simulink model "Droop_GC"  (Simulink 9.1)
settings: Solver=ode4  StartTime=0.0  StopTime=2.6  FixedStep=1e-6  RelTol=1e-3  EnableMultiTasking=on
InitFcn:
  | %% Circuit parameters
  | % LC filter
  | Lf_1 = 1.35e-3;
  | Rf_1 = 0.1;
  | Cf_1 = 50e-6;
  | 
  | Lf_2 = 1.35e-3;
  | Rf_2 = 0.1;
  | Cf_2 = 50e-6;
  | 
  | Lf_3 = 1.35e-3;
  | Rf_3 = 0.1;
  | Cf_3 = 50e-6;
  | 
  | % transmission line(grid coupling impedance)
  | L_1 = 0.35e-3;
  | R_1 = 0.03;
  | 
  | L_2 = 0.35e-3;
  | R_2 = 0.03;
  | 
  | L_3 = 0.35e-3;
  | R_3 = 0.03;
  | 
  | % Network
  | % active power loop
  | fn = 50;
  | wn = 2*pi*fn;
  | 
  | R_line_1 = 0.23;
  | L_line_1 = 0.1 / wn;
  | 
  | R_line_2 = 0.35;
  | L_line_2 = 0.58 / wn;
  | 
  | 
  | %% Control parameters
  | % power measurement LPF
  | wc = 31.41;
  | 
  | % Power droop
  | mp_1 = mp;
  | mp_2 = mp;
  | mp_3 = mp;
  | 
  | nq_1 = nq;
  | nq_2 = nq;
  | nq_3 = nq;
  | 
  | J1 = 0.1;
  | J2 = 0.1;
  | J3 = 0.1;
  | 
  | Pref_1 = Pref;
  | Pref_2 = Pref;
  | Pref_3 = Pref;
  | 
  | % outer voltage loop
  | Kpv_1 = 0.05;
  | Kiv_1 = 390;
  | ... (+76 lines)
values from neighbouring files (symbols this model uses):
  mp = 9.4e-5    (= 9.4e-05)    [model_coefficient.m]
  nq = 1.3e-3    (= 0.0013)    [model_coefficient.m]
  Pref = 10000    [model_coefficient.m]
  R1 = 25    [model_coefficient.m]
  R3 = 20    [model_coefficient.m]
libraries: powerlib x53, powerlib_meascontrol x25
(part 2 of 2)

== system Droop_GC/sm_computation/VSI 1/1_VSG control block/SRF PLL1 ==
  Vg_abc : Inport
  Demux2 : Demux  Outputs=3
  LPF2 : TransferFcn  Numerator=[wf_pll]  Denominator=[1 wf_pll]
  SRF_PLL : Subsystem
  Tclark : Subsystem
  Tpark : Subsystem
  Vg_theta : Outport
  wires:
  Demux2/1 -> Tclark/1(Ua)
  Demux2/2 -> Tclark/2(Ub)
  Demux2/3 -> Tclark/3(Uc)
  Tclark/1(Valpha) -> Tpark/1(Ualpha)
  Tpark/2(Uq) -> LPF2/1
  LPF2/1 -> SRF_PLL/1(vq)  "SRF_vq"
  Vg_abc/1 -> Demux2/1
  Tclark/2(Vbeta) -> Tpark/2(Ubeta)
  SRF_PLL/1(wt) -> Tpark/3(theta), Vg_theta/1  "SRF_wt_mod"

== system Droop_GC/sm_computation/VSI 1/1_VSG control block/Subsystem ==
  theta_g : Inport
  Enable_sync : Inport  Port=2
  theta_vsg : Inport  Port=3
  Add : Sum  Inputs=-+
  Constant : Constant  Value=0
  Gain : Gain  Gain=Kp_syn
  Gain1 : Gain  Gain=Ki_syn
  Integrator2 : Integrator
  Sum2 : Sum  Inputs=|++
  Switch : Switch  Criteria=u2 > Threshold
  delta_w : Outport
  wires:
  Gain1/1 -> Integrator2/1
  Integrator2/1 -> Sum2/2
  Sum2/1 -> Switch/1
  Add/1 -> Gain1/1, Gain/1
  Gain/1 -> Sum2/1
  theta_g/1 -> Add/2
  theta_vsg/1 -> Add/1
  Switch/1 -> delta_w/1
  Enable_sync/1 -> Switch/2
  Constant/1 -> Switch/3

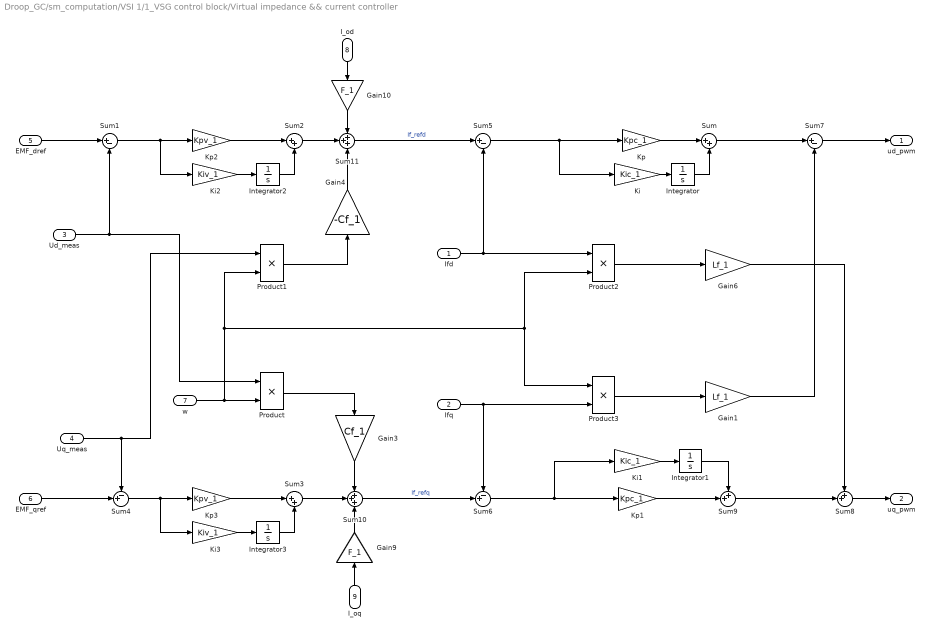
== system Droop_GC/sm_computation/VSI 1/1_VSG control block/Virtual impedance && current controller ==
  Ifd : Inport
  Ifq : Inport  Port=2
  Ud_meas : Inport  Port=3
  Uq_meas : Inport  Port=4
  EMF_dref : Inport  Port=5
  EMF_qref : Inport  Port=6
  w : Inport  Port=7
  I_od : Inport  Port=8
  I_oq : Inport  Port=9
  Gain1 : Gain  Gain=Lf_1
  Gain10 : Gain  Gain=F_1
  Gain3 : Gain  Gain=Cf_1
  Gain4 : Gain  Gain=-Cf_1
  Gain6 : Gain  Gain=Lf_1
  Gain9 : Gain  Gain=F_1
  Integrator{,1..3} (4 alike) : Integrator
  Ki : Gain  Gain=Kic_1
  Ki1 : Gain  Gain=Kic_1
  Ki2 : Gain  Gain=Kiv_1
  Ki3 : Gain  Gain=Kiv_1
  Kp : Gain  Gain=Kpc_1
  Kp1 : Gain  Gain=Kpc_1
  Kp2 : Gain  Gain=Kpv_1
  Kp3 : Gain  Gain=Kpv_1
  Product{,1..3} (4 alike) : Product
  Sum : Sum  Inputs=|++
  Sum1 : Sum  Inputs=|+-
  Sum10 : Sum  Inputs=+++
  Sum11 : Sum  Inputs=+++
  Sum2 : Sum  Inputs=|++
  Sum3 : Sum  Inputs=|++
  Sum4 : Sum  Inputs=-+|
  Sum5 : Sum  Inputs=|+-
  Sum6 : Sum  Inputs=-+|
  Sum7 : Sum  Inputs=|+-
  Sum8 : Sum  Inputs=++|
  Sum9 : Sum  Inputs=++|
  ud_pwm : Outport
  uq_pwm : Outport  Port=2
  wires:
  Sum7/1 -> ud_pwm/1
  Ifd/1 -> Sum5/2, Product2/1
  Ifq/1 -> Product3/2, Sum6/1
  Ki/1 -> Integrator/1
  Kp/1 -> Sum/1
  Integrator/1 -> Sum/2
  Sum11/1 -> Sum5/1  "If_refd"
  Sum10/1 -> Sum6/2  "If_refq"
  Sum8/1 -> uq_pwm/1
  Ki1/1 -> Integrator1/1
  Sum9/1 -> Sum8/2
  Sum5/1 -> Ki/1, Kp/1
  Kp1/1 -> Sum9/2
  Integrator1/1 -> Sum9/1
  Sum6/1 -> Ki1/1, Kp1/1
  EMF_dref/1 -> Sum1/1
  Ud_meas/1 -> Sum1/2, Product/1
  EMF_qref/1 -> Sum4/2
  Uq_meas/1 -> Product1/1, Sum4/1
  Sum1/1 -> Ki2/1, Kp2/1
  Integrator2/1 -> Sum2/2
  Kp2/1 -> Sum2/1
  Ki2/1 -> Integrator2/1
  Ki3/1 -> Integrator3/1
  Kp3/1 -> Sum3/1
  Sum4/1 -> Ki3/1, Kp3/1
  Integrator3/1 -> Sum3/2
  w/1 -> Product3/1, Product2/2, Product1/2, Product/2
  Product/1 -> Gain3/1
  Sum3/1 -> Sum10/2
  Gain3/1 -> Sum10/1
  Product1/1 -> Gain4/1
  Sum2/1 -> Sum11/2
  Gain4/1 -> Sum11/3
  I_oq/1 -> Gain9/1
  Gain9/1 -> Sum10/3
  I_od/1 -> Gain10/1
  Gain10/1 -> Sum11/1
  Sum/1 -> Sum7/1
  Product2/1 -> Gain6/1
  Gain6/1 -> Sum8/1
  Product3/1 -> Gain1/1
  Gain1/1 -> Sum7/2

== system Droop_GC/sm_computation/VSI 1/1_VSG control block/active power controller ==
  Pe : Inport
  delta_w : Inport  Port=2
  Constant : Constant  Value=wn
  Gain2 : Gain  Gain=mp_1
  Integrator3 : Integrator
  Pref_INV1 : Constant  Value=Pref_1
  Sum2 : Sum  Inputs=|++
  Sum3 : Sum  Inputs=+-
  Sum6 : Sum  Inputs=++|
  theta : Outport
  w : Outport  Port=2
  wires:
  Pe/1 -> Sum3/2
  Pref_INV1/1 -> Sum3/1
  Sum3/1 -> Gain2/1
  Constant/1 -> Sum6/2
  Gain2/1 -> Sum6/1
  delta_w/1 -> Sum2/2
  Sum6/1 -> Sum2/1  "w"
  Sum2/1 -> w/1, Integrator3/1
  Integrator3/1 -> theta/1

== system Droop_GC/sm_computation/VSI 1/1_VSG control block/reactive power controller ==
  Qe : Inport
  Dq_1 : Gain  Gain=nq_1
  Sum1 : Sum  Inputs=|+-
  Vn1 : Constant  Value=sqrt(2)*V_phase_rms
  Em : Outport
  wires:
  Sum1/1 -> Em/1  "delta_P"
  Qe/1 -> Dq_1/1
  Dq_1/1 -> Sum1/2
  Vn1/1 -> Sum1/1

== system Droop_GC/sm_computation/VSI 2/1_VSG control block/Power Calculation ==
  note: Iabc
  note: Vabc
  Vin : Inport
  Iin : Inport  Port=2
  Add : Sum
  Add1 : Sum  Inputs=-+
  Demux1 : Demux  Outputs=3
  Demux2 : Demux  Outputs=3
  Gain1 : Gain  Gain=3/2
  Gain2 : Gain  Gain=3/2
  Product{,1..3} (4 alike) : Product
  Terminator : Terminator
  Terminator1 : Terminator
  abc to Alpha-Beta-Zero : powerlib_meascontrol/Transformations/abc to Alpha-Beta-Zero
      settings: SourceProductName=Simscape Power Systems
  abc to Alpha-Beta-Zero1 : powerlib_meascontrol/Transformations/abc to Alpha-Beta-Zero
      settings: SourceProductName=Simscape Power Systems
  P : Outport
  Q : Outport  Port=2
  wires:
  Add1/1 -> Gain1/1
  Add/1 -> Gain2/1
  Demux2/2 -> Product1/2, Product2/2
  Product3/1 -> Add1/2
  Product2/1 -> Add1/1
  Product1/1 -> Add/2
  Product/1 -> Add/1
  abc to Alpha-Beta-Zero/1 -> Demux1/1
  Demux1/1 -> Product2/1, Product/1
  abc to Alpha-Beta-Zero1/1 -> Demux2/1
  Demux2/3 -> Terminator1/1
  Demux1/3 -> Terminator/1
  Demux2/1 -> Product3/2, Product/2
  Demux1/2 -> Product3/1, Product1/1
  Vin/1 -> abc to Alpha-Beta-Zero/1
  Iin/1 -> abc to Alpha-Beta-Zero1/1
  Gain2/1 -> P/1
  Gain1/1 -> Q/1

== system Droop_GC/sm_computation/VSI 2/1_VSG control block/SRF PLL ==
  Vg_abc : Inport
  Demux2 : Demux  Outputs=3
  LPF2 : TransferFcn  Numerator=[wf_pll]  Denominator=[1 wf_pll]
  LPF3 : TransferFcn  Numerator=[wf_pll]  Denominator=[1 wf_pll]
  SRF_PLL : Subsystem
  Tclark : Subsystem
  Tpark : Subsystem
  Vg_theta : Outport
  wires:
  Demux2/1 -> Tclark/1(Ua)
  Demux2/2 -> Tclark/2(Ub)
  Demux2/3 -> Tclark/3(Uc)
  Tpark/1(Ud) -> LPF3/1
  Tclark/1(Valpha) -> Tpark/1(Ualpha)
  Tpark/2(Uq) -> LPF2/1
  LPF2/1 -> SRF_PLL/1(vq)  "SRF_vq"
  Vg_abc/1 -> Demux2/1
  Tclark/2(Vbeta) -> Tpark/2(Ubeta)
  SRF_PLL/1(wt) -> Tpark/3(theta), Vg_theta/1  "SRF_wt_mod"

== system Droop_GC/sm_computation/VSI 2/1_VSG control block/SRF PLL1 ==
  Vg_abc : Inport
  Demux2 : Demux  Outputs=3
  LPF2 : TransferFcn  Numerator=[wf_pll]  Denominator=[1 wf_pll]
  SRF_PLL : Subsystem
  Tclark : Subsystem
  Tpark : Subsystem
  Vg_theta : Outport
  wires:
  Demux2/1 -> Tclark/1(Ua)
  Demux2/2 -> Tclark/2(Ub)
  Demux2/3 -> Tclark/3(Uc)
  Tclark/1(Valpha) -> Tpark/1(Ualpha)
  Tpark/2(Uq) -> LPF2/1
  LPF2/1 -> SRF_PLL/1(vq)  "SRF_vq"
  Vg_abc/1 -> Demux2/1
  Tclark/2(Vbeta) -> Tpark/2(Ubeta)
  SRF_PLL/1(wt) -> Tpark/3(theta), Vg_theta/1  "SRF_wt_mod"

== system Droop_GC/sm_computation/VSI 2/1_VSG control block/Subsystem ==
  theta_g : Inport
  Enable_sync : Inport  Port=2
  theta_vsg : Inport  Port=3
  Add : Sum  Inputs=-+
  Constant : Constant  Value=0
  Gain : Gain  Gain=Kp_syn
  Gain1 : Gain  Gain=Ki_syn
  Integrator2 : Integrator
  Sum2 : Sum  Inputs=|++
  Switch : Switch  Criteria=u2 > Threshold
  delta_w : Outport
  wires:
  Gain1/1 -> Integrator2/1
  Integrator2/1 -> Sum2/2
  Sum2/1 -> Switch/1
  Add/1 -> Gain1/1, Gain/1
  Gain/1 -> Sum2/1
  theta_g/1 -> Add/2
  theta_vsg/1 -> Add/1
  Switch/1 -> delta_w/1
  Enable_sync/1 -> Switch/2
  Constant/1 -> Switch/3

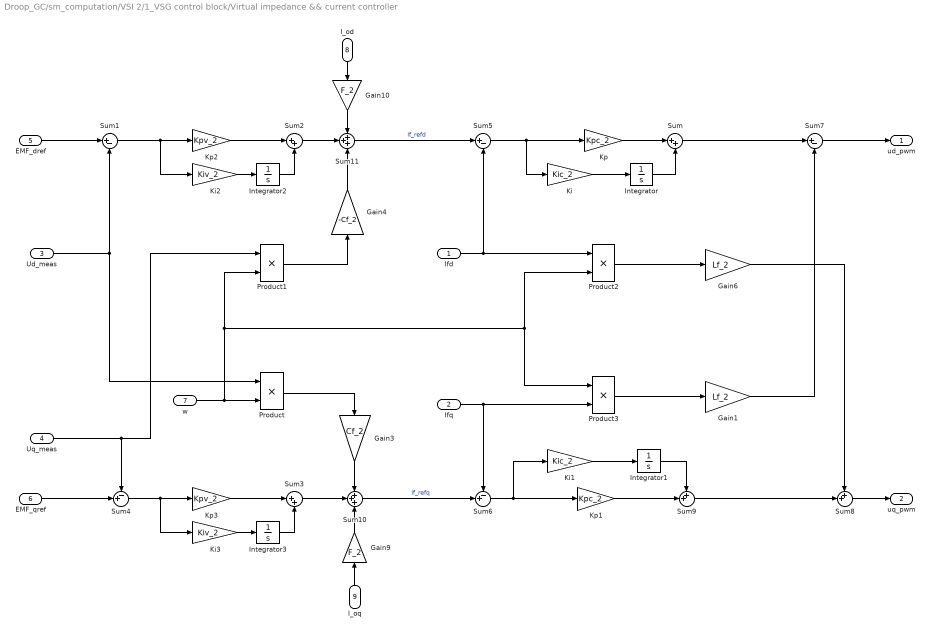
== system Droop_GC/sm_computation/VSI 2/1_VSG control block/Virtual impedance && current controller ==
  Ifd : Inport
  Ifq : Inport  Port=2
  Ud_meas : Inport  Port=3
  Uq_meas : Inport  Port=4
  EMF_dref : Inport  Port=5
  EMF_qref : Inport  Port=6
  w : Inport  Port=7
  I_od : Inport  Port=8
  I_oq : Inport  Port=9
  Gain1 : Gain  Gain=Lf_2
  Gain10 : Gain  Gain=F_2
  Gain3 : Gain  Gain=Cf_2
  Gain4 : Gain  Gain=-Cf_2
  Gain6 : Gain  Gain=Lf_2
  Gain9 : Gain  Gain=F_2
  Integrator{,1..3} (4 alike) : Integrator
  Ki : Gain  Gain=Kic_2
  Ki1 : Gain  Gain=Kic_2
  Ki2 : Gain  Gain=Kiv_2
  Ki3 : Gain  Gain=Kiv_2
  Kp : Gain  Gain=Kpc_2
  Kp1 : Gain  Gain=Kpc_2
  Kp2 : Gain  Gain=Kpv_2
  Kp3 : Gain  Gain=Kpv_2
  Product{,1..3} (4 alike) : Product
  Sum : Sum  Inputs=|++
  Sum1 : Sum  Inputs=|+-
  Sum10 : Sum  Inputs=+++
  Sum11 : Sum  Inputs=+++
  Sum2 : Sum  Inputs=|++
  Sum3 : Sum  Inputs=|++
  Sum4 : Sum  Inputs=-+|
  Sum5 : Sum  Inputs=|+-
  Sum6 : Sum  Inputs=-+|
  Sum7 : Sum  Inputs=|+-
  Sum8 : Sum  Inputs=++|
  Sum9 : Sum  Inputs=++|
  ud_pwm : Outport
  uq_pwm : Outport  Port=2
  wires:
  Gain1/1 -> Sum7/2
  Product3/1 -> Gain1/1
  Gain6/1 -> Sum8/1
  Product2/1 -> Gain6/1
  Sum/1 -> Sum7/1
  Gain10/1 -> Sum11/1
  I_od/1 -> Gain10/1
  Gain9/1 -> Sum10/3
  I_oq/1 -> Gain9/1
  Gain4/1 -> Sum11/3
  Sum2/1 -> Sum11/2
  Product1/1 -> Gain4/1
  Gain3/1 -> Sum10/1
  Sum3/1 -> Sum10/2
  Product/1 -> Gain3/1
  w/1 -> Product/2, Product1/2, Product2/2, Product3/1
  Integrator3/1 -> Sum3/2
  Sum4/1 -> Kp3/1, Ki3/1
  Kp3/1 -> Sum3/1
  Ki3/1 -> Integrator3/1
  Ki2/1 -> Integrator2/1
  Kp2/1 -> Sum2/1
  Integrator2/1 -> Sum2/2
  Sum1/1 -> Kp2/1, Ki2/1
  Uq_meas/1 -> Product1/1, Sum4/1
  EMF_qref/1 -> Sum4/2
  Ud_meas/1 -> Product/1, Sum1/2
  EMF_dref/1 -> Sum1/1
  Sum6/1 -> Kp1/1, Ki1/1
  Integrator1/1 -> Sum9/1
  Kp1/1 -> Sum9/2
  Sum5/1 -> Kp/1, Ki/1
  Sum9/1 -> Sum8/2
  Ki1/1 -> Integrator1/1
  Sum8/1 -> uq_pwm/1
  Sum10/1 -> Sum6/2  "If_refq"
  Sum11/1 -> Sum5/1  "If_refd"
  Integrator/1 -> Sum/2
  Kp/1 -> Sum/1
  Ki/1 -> Integrator/1
  Ifq/1 -> Sum6/1, Product3/2
  Ifd/1 -> Product2/1, Sum5/2
  Sum7/1 -> ud_pwm/1

== system Droop_GC/sm_computation/VSI 2/1_VSG control block/active power controller ==
  Pe : Inport
  delta_w : Inport  Port=2
  Constant : Constant  Value=wn
  Gain1 : Gain  Gain=mp_2
  Integrator1 : Integrator
  Pref_INV2 : Constant  Value=Pref_2
  Sum1 : Sum  Inputs=++|
  Sum2 : Sum  Inputs=|++
  Sum3 : Sum  Inputs=|+-
  theta : Outport
  w : Outport  Port=2
  wires:
  Pref_INV2/1 -> Sum3/1
  Pe/1 -> Sum3/2
  Integrator1/1 -> theta/1
  delta_w/1 -> Sum2/2
  Sum2/1 -> w/1, Integrator1/1
  Sum3/1 -> Gain1/1
  Gain1/1 -> Sum1/1
  Constant/1 -> Sum1/2
  Sum1/1 -> Sum2/1

== system Droop_GC/sm_computation/VSI 2/1_VSG control block/reactive power controller ==
  Qe : Inport
  Dq_2 : Gain  Gain=nq_2
  Sum1 : Sum  Inputs=|+-
  Vn1 : Constant  Value=sqrt(2)*V_phase_rms
  Em : Outport
  wires:
  Vn1/1 -> Sum1/1
  Dq_2/1 -> Sum1/2
  Qe/1 -> Dq_2/1
  Sum1/1 -> Em/1  "delta_P"

== system Droop_GC/sm_computation/VSI 3/1_VSG control block/Power Calculation ==
  note: Iabc
  note: Vabc
  Vin : Inport
  Iin : Inport  Port=2
  Add : Sum
  Add1 : Sum  Inputs=-+
  Demux1 : Demux  Outputs=3
  Demux2 : Demux  Outputs=3
  Gain1 : Gain  Gain=3/2
  Gain2 : Gain  Gain=3/2
  Product{,1..3} (4 alike) : Product
  Terminator : Terminator
  Terminator1 : Terminator
  abc to Alpha-Beta-Zero : powerlib_meascontrol/Transformations/abc to Alpha-Beta-Zero
      settings: SourceProductName=Simscape Power Systems
  abc to Alpha-Beta-Zero1 : powerlib_meascontrol/Transformations/abc to Alpha-Beta-Zero
      settings: SourceProductName=Simscape Power Systems
  P : Outport
  Q : Outport  Port=2
  wires:
  Add1/1 -> Gain1/1
  Add/1 -> Gain2/1
  Demux2/2 -> Product1/2, Product2/2
  Product3/1 -> Add1/2
  Product2/1 -> Add1/1
  Product1/1 -> Add/2
  Product/1 -> Add/1
  abc to Alpha-Beta-Zero/1 -> Demux1/1
  Demux1/1 -> Product2/1, Product/1
  abc to Alpha-Beta-Zero1/1 -> Demux2/1
  Demux2/3 -> Terminator1/1
  Demux1/3 -> Terminator/1
  Demux2/1 -> Product3/2, Product/2
  Demux1/2 -> Product3/1, Product1/1
  Vin/1 -> abc to Alpha-Beta-Zero/1
  Iin/1 -> abc to Alpha-Beta-Zero1/1
  Gain2/1 -> P/1
  Gain1/1 -> Q/1

== system Droop_GC/sm_computation/VSI 3/1_VSG control block/SRF PLL ==
  Vg_abc : Inport
  Demux2 : Demux  Outputs=3
  LPF2 : TransferFcn  Numerator=[wf_pll]  Denominator=[1 wf_pll]
  LPF3 : TransferFcn  Numerator=[wf_pll]  Denominator=[1 wf_pll]
  SRF_PLL : Subsystem
  Tclark : Subsystem
  Tpark : Subsystem
  Vg_theta : Outport
  wires:
  Demux2/1 -> Tclark/1(Ua)
  Demux2/2 -> Tclark/2(Ub)
  Demux2/3 -> Tclark/3(Uc)
  Tpark/1(Ud) -> LPF3/1
  Tclark/1(Valpha) -> Tpark/1(Ualpha)
  Tpark/2(Uq) -> LPF2/1
  LPF2/1 -> SRF_PLL/1(vq)  "SRF_vq"
  Vg_abc/1 -> Demux2/1
  Tclark/2(Vbeta) -> Tpark/2(Ubeta)
  SRF_PLL/1(wt) -> Tpark/3(theta), Vg_theta/1  "SRF_wt_mod"

== system Droop_GC/sm_computation/VSI 3/1_VSG control block/SRF PLL1 ==
  Vg_abc : Inport
  Demux2 : Demux  Outputs=3
  LPF2 : TransferFcn  Numerator=[wf_pll]  Denominator=[1 wf_pll]
  SRF_PLL : Subsystem
  Tclark : Subsystem
  Tpark : Subsystem
  Vg_theta : Outport
  wires:
  Demux2/1 -> Tclark/1(Ua)
  Demux2/2 -> Tclark/2(Ub)
  Demux2/3 -> Tclark/3(Uc)
  Tclark/1(Valpha) -> Tpark/1(Ualpha)
  Tpark/2(Uq) -> LPF2/1
  LPF2/1 -> SRF_PLL/1(vq)  "SRF_vq"
  Vg_abc/1 -> Demux2/1
  Tclark/2(Vbeta) -> Tpark/2(Ubeta)
  SRF_PLL/1(wt) -> Tpark/3(theta), Vg_theta/1  "SRF_wt_mod"

== system Droop_GC/sm_computation/VSI 3/1_VSG control block/Subsystem ==
  theta_g : Inport
  Enable_sync : Inport  Port=2
  theta_vsg : Inport  Port=3
  Add : Sum  Inputs=-+
  Constant : Constant  Value=0
  Gain : Gain  Gain=Kp_syn
  Gain1 : Gain  Gain=Ki_syn
  Integrator2 : Integrator
  Sum2 : Sum  Inputs=|++
  Switch : Switch  Criteria=u2 > Threshold
  delta_w : Outport
  wires:
  Gain1/1 -> Integrator2/1
  Integrator2/1 -> Sum2/2
  Sum2/1 -> Switch/1
  Add/1 -> Gain1/1, Gain/1
  Gain/1 -> Sum2/1
  theta_g/1 -> Add/2
  theta_vsg/1 -> Add/1
  Switch/1 -> delta_w/1
  Enable_sync/1 -> Switch/2
  Constant/1 -> Switch/3

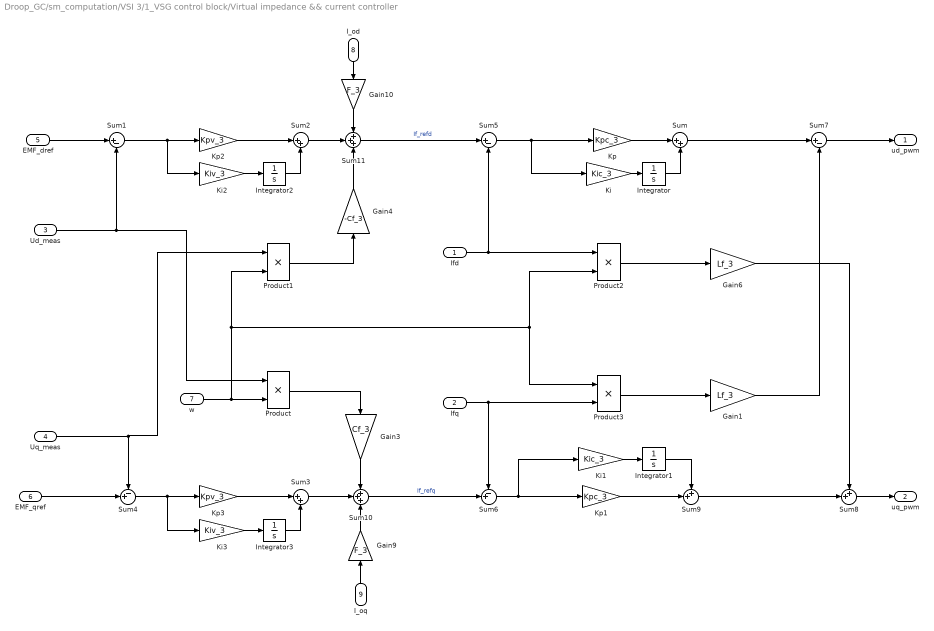
== system Droop_GC/sm_computation/VSI 3/1_VSG control block/Virtual impedance && current controller ==
  Ifd : Inport
  Ifq : Inport  Port=2
  Ud_meas : Inport  Port=3
  Uq_meas : Inport  Port=4
  EMF_dref : Inport  Port=5
  EMF_qref : Inport  Port=6
  w : Inport  Port=7
  I_od : Inport  Port=8
  I_oq : Inport  Port=9
  Gain1 : Gain  Gain=Lf_3
  Gain10 : Gain  Gain=F_3
  Gain3 : Gain  Gain=Cf_3
  Gain4 : Gain  Gain=-Cf_3
  Gain6 : Gain  Gain=Lf_3
  Gain9 : Gain  Gain=F_3
  Integrator{,1..3} (4 alike) : Integrator
  Ki : Gain  Gain=Kic_3
  Ki1 : Gain  Gain=Kic_3
  Ki2 : Gain  Gain=Kiv_3
  Ki3 : Gain  Gain=Kiv_3
  Kp : Gain  Gain=Kpc_3
  Kp1 : Gain  Gain=Kpc_3
  Kp2 : Gain  Gain=Kpv_3
  Kp3 : Gain  Gain=Kpv_3
  Product{,1..3} (4 alike) : Product
  Sum : Sum  Inputs=|++
  Sum1 : Sum  Inputs=|+-
  Sum10 : Sum  Inputs=+++
  Sum11 : Sum  Inputs=+++
  Sum2 : Sum  Inputs=|++
  Sum3 : Sum  Inputs=|++
  Sum4 : Sum  Inputs=-+|
  Sum5 : Sum  Inputs=|+-
  Sum6 : Sum  Inputs=-+|
  Sum7 : Sum  Inputs=|+-
  Sum8 : Sum  Inputs=++|
  Sum9 : Sum  Inputs=++|
  ud_pwm : Outport
  uq_pwm : Outport  Port=2
  wires:
  Sum7/1 -> ud_pwm/1
  Ifd/1 -> Sum5/2, Product2/1
  Ifq/1 -> Product3/2, Sum6/1
  Ki/1 -> Integrator/1
  Kp/1 -> Sum/1
  Integrator/1 -> Sum/2
  Sum11/1 -> Sum5/1  "If_refd"
  Sum10/1 -> Sum6/2  "If_refq"
  Sum8/1 -> uq_pwm/1
  Ki1/1 -> Integrator1/1
  Sum9/1 -> Sum8/2
  Sum5/1 -> Ki/1, Kp/1
  Kp1/1 -> Sum9/2
  Integrator1/1 -> Sum9/1
  Sum6/1 -> Ki1/1, Kp1/1
  EMF_dref/1 -> Sum1/1
  Ud_meas/1 -> Sum1/2, Product/1
  EMF_qref/1 -> Sum4/2
  Uq_meas/1 -> Product1/1, Sum4/1
  Sum1/1 -> Ki2/1, Kp2/1
  Integrator2/1 -> Sum2/2
  Kp2/1 -> Sum2/1
  Ki2/1 -> Integrator2/1
  Ki3/1 -> Integrator3/1
  Kp3/1 -> Sum3/1
  Sum4/1 -> Ki3/1, Kp3/1
  Integrator3/1 -> Sum3/2
  w/1 -> Product3/1, Product2/2, Product1/2, Product/2
  Product/1 -> Gain3/1
  Sum3/1 -> Sum10/2
  Gain3/1 -> Sum10/1
  Product1/1 -> Gain4/1
  Sum2/1 -> Sum11/2
  Gain4/1 -> Sum11/3
  I_oq/1 -> Gain9/1
  Gain9/1 -> Sum10/3
  I_od/1 -> Gain10/1
  Gain10/1 -> Sum11/1
  Sum/1 -> Sum7/1
  Product2/1 -> Gain6/1
  Gain6/1 -> Sum8/1
  Product3/1 -> Gain1/1
  Gain1/1 -> Sum7/2

== system Droop_GC/sm_computation/VSI 3/1_VSG control block/active power controller ==
  Pe : Inport
  delta_w : Inport  Port=2
  Constant : Constant  Value=wn
  Gain1 : Gain  Gain=mp_3
  Integrator1 : Integrator
  Pref_INV3 : Constant  Value=Pref_3
  Sum1 : Sum  Inputs=++|
  Sum2 : Sum  Inputs=|+-
  Sum3 : Sum  Inputs=|++
  theta : Outport
  w : Outport  Port=2
  wires:
  Pe/1 -> Sum2/2
  Pref_INV3/1 -> Sum2/1
  Integrator1/1 -> theta/1
  delta_w/1 -> Sum3/2
  Sum3/1 -> w/1, Integrator1/1
  Sum2/1 -> Gain1/1
  Constant/1 -> Sum1/2
  Gain1/1 -> Sum1/1
  Sum1/1 -> Sum3/1  "w"

== system Droop_GC/sm_computation/VSI 3/1_VSG control block/reactive power controller ==
  Qe : Inport
  Dq_3 : Gain  Gain=nq_3
  Sum1 : Sum  Inputs=|+-
  Vn1 : Constant  Value=sqrt(2)*V_phase_rms
  Em : Outport
  wires:
  Sum1/1 -> Em/1  "delta_P"
  Qe/1 -> Dq_3/1
  Dq_3/1 -> Sum1/2
  Vn1/1 -> Sum1/1

== system Droop_GC/sm_computation/VSI 1/1_VSG control block/SRF PLL/SRF_PLL ==
  vq : Inport
  Center_Fre : Constant  Value=wn
  Center_Fre1 : Constant  Value=220*sqrt(2)
  Divide : Product  Inputs=*/
  Integrator : Integrator
  Integrator1 : Integrator
  Ki : Gain  Gain=Ki_pll
  Kp : Gain  Gain=Kp_pll
  Sum : Sum  Inputs=|++
  Sum1 : Sum  Inputs=++|
  wt : Outport
  wires:
  Divide/1 -> Ki/1, Kp/1
  Kp/1 -> Sum/1
  Ki/1 -> Integrator/1
  Integrator/1 -> Sum/2
  Sum/1 -> Sum1/2
  Sum1/1 -> Integrator1/1
  Integrator1/1 -> wt/1
  vq/1 -> Divide/1
  Center_Fre/1 -> Sum1/1
  Center_Fre1/1 -> Divide/2

== system Droop_GC/sm_computation/VSI 1/1_VSG control block/SRF PLL/Tclark ==
  Ua : Inport
  Ub : Inport  Port=2
  Uc : Inport  Port=3
  Constant : Constant  Value=2/3
  Constant1 : Constant  Value=-1/3
  Constant2 : Constant  Value=-1/3
  Constant3 : Constant  Value=1/sqrt(3)
  Constant4 : Constant  Value=-1/sqrt(3)
  Product{,1..4} (5 alike) : Product
  Sum : Sum  Inputs=+++
  Sum1 : Sum
  Valpha : Outport
  Vbeta : Outport  Port=2
  wires:
  Product/1 -> Sum/1
  Constant1/1 -> Product1/1
  Product2/1 -> Sum/3
  Ua/1 -> Product/2
  Constant4/1 -> Product4/2
  Constant2/1 -> Product2/1
  Uc/1 -> Product4/1, Product2/2
  Constant/1 -> Product/1
  Sum/1 -> Valpha/1
  Product1/1 -> Sum/2
  Constant3/1 -> Product3/2
  Sum1/1 -> Vbeta/1
  Product3/1 -> Sum1/1
  Product4/1 -> Sum1/2
  Ub/1 -> Product3/1, Product1/2

== system Droop_GC/sm_computation/VSI 1/1_VSG control block/SRF PLL/Tpark ==
  Ualpha : Inport
  Ubeta : Inport  Port=2
  theta : Inport  Port=3
  Product{,1..3} (4 alike) : Product
  Sum : Sum
  Sum1 : Sum  Inputs=-+
  Trigonometric Function : Trigonometry
  Trigonometric Function1 : Trigonometry  Operator=cos
  Ud : Outport
  Uq : Outport  Port=2
  wires:
  Ualpha/1 -> Product/1, Product3/1
  Product3/1 -> Sum1/1
  Product1/1 -> Sum/2
  Trigonometric Function1/1 -> Product2/2, Product/2
  Ubeta/1 -> Product1/1, Product2/1
  Sum/1 -> Ud/1
  Product/1 -> Sum/1
  Trigonometric Function/1 -> Product3/2, Product1/2
  Sum1/1 -> Uq/1
  theta/1 -> Trigonometric Function1/1, Trigonometric Function/1
  Product2/1 -> Sum1/2

== system Droop_GC/sm_computation/VSI 1/1_VSG control block/SRF PLL1/SRF_PLL ==
  vq : Inport
  Center_Fre : Constant  Value=wn
  Center_Fre1 : Constant  Value=220*sqrt(2)
  Divide : Product  Inputs=*/
  Integrator : Integrator
  Integrator1 : Integrator
  Ki : Gain  Gain=Ki_pll
  Kp : Gain  Gain=Kp_pll
  Sum : Sum  Inputs=|++
  Sum1 : Sum  Inputs=++|
  wt : Outport
  wires:
  Divide/1 -> Ki/1, Kp/1
  Kp/1 -> Sum/1
  Ki/1 -> Integrator/1
  Integrator/1 -> Sum/2
  Sum/1 -> Sum1/2
  Sum1/1 -> Integrator1/1
  Integrator1/1 -> wt/1
  vq/1 -> Divide/1
  Center_Fre/1 -> Sum1/1
  Center_Fre1/1 -> Divide/2

== system Droop_GC/sm_computation/VSI 1/1_VSG control block/SRF PLL1/Tclark ==
  Ua : Inport
  Ub : Inport  Port=2
  Uc : Inport  Port=3
  Constant : Constant  Value=2/3
  Constant1 : Constant  Value=-1/3
  Constant2 : Constant  Value=-1/3
  Constant3 : Constant  Value=1/sqrt(3)
  Constant4 : Constant  Value=-1/sqrt(3)
  Product{,1..4} (5 alike) : Product
  Sum : Sum  Inputs=+++
  Sum1 : Sum
  Valpha : Outport
  Vbeta : Outport  Port=2
  wires:
  Product/1 -> Sum/1
  Constant1/1 -> Product1/1
  Product2/1 -> Sum/3
  Ua/1 -> Product/2
  Constant4/1 -> Product4/2
  Constant2/1 -> Product2/1
  Uc/1 -> Product4/1, Product2/2
  Constant/1 -> Product/1
  Sum/1 -> Valpha/1
  Product1/1 -> Sum/2
  Constant3/1 -> Product3/2
  Sum1/1 -> Vbeta/1
  Product3/1 -> Sum1/1
  Product4/1 -> Sum1/2
  Ub/1 -> Product3/1, Product1/2

== system Droop_GC/sm_computation/VSI 1/1_VSG control block/SRF PLL1/Tpark ==
  Ualpha : Inport
  Ubeta : Inport  Port=2
  theta : Inport  Port=3
  Product{,1..3} (4 alike) : Product
  Sum : Sum
  Sum1 : Sum  Inputs=-+
  Trigonometric Function : Trigonometry
  Trigonometric Function1 : Trigonometry  Operator=cos
  Ud : Outport
  Uq : Outport  Port=2
  wires:
  Ualpha/1 -> Product/1, Product3/1
  Product3/1 -> Sum1/1
  Product1/1 -> Sum/2
  Trigonometric Function1/1 -> Product2/2, Product/2
  Ubeta/1 -> Product1/1, Product2/1
  Sum/1 -> Ud/1
  Product/1 -> Sum/1
  Trigonometric Function/1 -> Product3/2, Product1/2
  Sum1/1 -> Uq/1
  theta/1 -> Trigonometric Function1/1, Trigonometric Function/1
  Product2/1 -> Sum1/2

== system Droop_GC/sm_computation/VSI 2/1_VSG control block/SRF PLL/SRF_PLL ==
  vq : Inport
  Center_Fre : Constant  Value=wn
  Center_Fre1 : Constant  Value=220*sqrt(2)
  Divide : Product  Inputs=*/
  Integrator : Integrator
  Integrator1 : Integrator
  Ki : Gain  Gain=Ki_pll
  Kp : Gain  Gain=Kp_pll
  Sum : Sum  Inputs=|++
  Sum1 : Sum  Inputs=++|
  wt : Outport
  wires:
  Divide/1 -> Ki/1, Kp/1
  Kp/1 -> Sum/1
  Ki/1 -> Integrator/1
  Integrator/1 -> Sum/2
  Sum/1 -> Sum1/2
  Sum1/1 -> Integrator1/1
  Integrator1/1 -> wt/1
  vq/1 -> Divide/1
  Center_Fre/1 -> Sum1/1
  Center_Fre1/1 -> Divide/2

== system Droop_GC/sm_computation/VSI 2/1_VSG control block/SRF PLL/Tclark ==
  Ua : Inport
  Ub : Inport  Port=2
  Uc : Inport  Port=3
  Constant : Constant  Value=2/3
  Constant1 : Constant  Value=-1/3
  Constant2 : Constant  Value=-1/3
  Constant3 : Constant  Value=1/sqrt(3)
  Constant4 : Constant  Value=-1/sqrt(3)
  Product{,1..4} (5 alike) : Product
  Sum : Sum  Inputs=+++
  Sum1 : Sum
  Valpha : Outport
  Vbeta : Outport  Port=2
  wires:
  Product/1 -> Sum/1
  Constant1/1 -> Product1/1
  Product2/1 -> Sum/3
  Ua/1 -> Product/2
  Constant4/1 -> Product4/2
  Constant2/1 -> Product2/1
  Uc/1 -> Product4/1, Product2/2
  Constant/1 -> Product/1
  Sum/1 -> Valpha/1
  Product1/1 -> Sum/2
  Constant3/1 -> Product3/2
  Sum1/1 -> Vbeta/1
  Product3/1 -> Sum1/1
  Product4/1 -> Sum1/2
  Ub/1 -> Product3/1, Product1/2

== system Droop_GC/sm_computation/VSI 2/1_VSG control block/SRF PLL/Tpark ==
  Ualpha : Inport
  Ubeta : Inport  Port=2
  theta : Inport  Port=3
  Product{,1..3} (4 alike) : Product
  Sum : Sum
  Sum1 : Sum  Inputs=-+
  Trigonometric Function : Trigonometry
  Trigonometric Function1 : Trigonometry  Operator=cos
  Ud : Outport
  Uq : Outport  Port=2
  wires:
  Ualpha/1 -> Product/1, Product3/1
  Product3/1 -> Sum1/1
  Product1/1 -> Sum/2
  Trigonometric Function1/1 -> Product2/2, Product/2
  Ubeta/1 -> Product1/1, Product2/1
  Sum/1 -> Ud/1
  Product/1 -> Sum/1
  Trigonometric Function/1 -> Product3/2, Product1/2
  Sum1/1 -> Uq/1
  theta/1 -> Trigonometric Function1/1, Trigonometric Function/1
  Product2/1 -> Sum1/2

== system Droop_GC/sm_computation/VSI 2/1_VSG control block/SRF PLL1/SRF_PLL ==
  vq : Inport
  Center_Fre : Constant  Value=wn
  Center_Fre1 : Constant  Value=220*sqrt(2)
  Divide : Product  Inputs=*/
  Integrator : Integrator
  Integrator1 : Integrator
  Ki : Gain  Gain=Ki_pll
  Kp : Gain  Gain=Kp_pll
  Sum : Sum  Inputs=|++
  Sum1 : Sum  Inputs=++|
  wt : Outport
  wires:
  Divide/1 -> Ki/1, Kp/1
  Kp/1 -> Sum/1
  Ki/1 -> Integrator/1
  Integrator/1 -> Sum/2
  Sum/1 -> Sum1/2
  Sum1/1 -> Integrator1/1
  Integrator1/1 -> wt/1
  vq/1 -> Divide/1
  Center_Fre/1 -> Sum1/1
  Center_Fre1/1 -> Divide/2

== system Droop_GC/sm_computation/VSI 2/1_VSG control block/SRF PLL1/Tclark ==
  Ua : Inport
  Ub : Inport  Port=2
  Uc : Inport  Port=3
  Constant : Constant  Value=2/3
  Constant1 : Constant  Value=-1/3
  Constant2 : Constant  Value=-1/3
  Constant3 : Constant  Value=1/sqrt(3)
  Constant4 : Constant  Value=-1/sqrt(3)
  Product{,1..4} (5 alike) : Product
  Sum : Sum  Inputs=+++
  Sum1 : Sum
  Valpha : Outport
  Vbeta : Outport  Port=2
  wires:
  Product/1 -> Sum/1
  Constant1/1 -> Product1/1
  Product2/1 -> Sum/3
  Ua/1 -> Product/2
  Constant4/1 -> Product4/2
  Constant2/1 -> Product2/1
  Uc/1 -> Product4/1, Product2/2
  Constant/1 -> Product/1
  Sum/1 -> Valpha/1
  Product1/1 -> Sum/2
  Constant3/1 -> Product3/2
  Sum1/1 -> Vbeta/1
  Product3/1 -> Sum1/1
  Product4/1 -> Sum1/2
  Ub/1 -> Product3/1, Product1/2

== system Droop_GC/sm_computation/VSI 2/1_VSG control block/SRF PLL1/Tpark ==
  Ualpha : Inport
  Ubeta : Inport  Port=2
  theta : Inport  Port=3
  Product{,1..3} (4 alike) : Product
  Sum : Sum
  Sum1 : Sum  Inputs=-+
  Trigonometric Function : Trigonometry
  Trigonometric Function1 : Trigonometry  Operator=cos
  Ud : Outport
  Uq : Outport  Port=2
  wires:
  Ualpha/1 -> Product/1, Product3/1
  Product3/1 -> Sum1/1
  Product1/1 -> Sum/2
  Trigonometric Function1/1 -> Product2/2, Product/2
  Ubeta/1 -> Product1/1, Product2/1
  Sum/1 -> Ud/1
  Product/1 -> Sum/1
  Trigonometric Function/1 -> Product3/2, Product1/2
  Sum1/1 -> Uq/1
  theta/1 -> Trigonometric Function1/1, Trigonometric Function/1
  Product2/1 -> Sum1/2

== system Droop_GC/sm_computation/VSI 3/1_VSG control block/SRF PLL/SRF_PLL ==
  vq : Inport
  Center_Fre : Constant  Value=wn
  Center_Fre1 : Constant  Value=220*sqrt(2)
  Divide : Product  Inputs=*/
  Integrator : Integrator
  Integrator1 : Integrator
  Ki : Gain  Gain=Ki_pll
  Kp : Gain  Gain=Kp_pll
  Sum : Sum  Inputs=|++
  Sum1 : Sum  Inputs=++|
  wt : Outport
  wires:
  Divide/1 -> Ki/1, Kp/1
  Kp/1 -> Sum/1
  Ki/1 -> Integrator/1
  Integrator/1 -> Sum/2
  Sum/1 -> Sum1/2
  Sum1/1 -> Integrator1/1
  Integrator1/1 -> wt/1
  vq/1 -> Divide/1
  Center_Fre/1 -> Sum1/1
  Center_Fre1/1 -> Divide/2

== system Droop_GC/sm_computation/VSI 3/1_VSG control block/SRF PLL/Tclark ==
  Ua : Inport
  Ub : Inport  Port=2
  Uc : Inport  Port=3
  Constant : Constant  Value=2/3
  Constant1 : Constant  Value=-1/3
  Constant2 : Constant  Value=-1/3
  Constant3 : Constant  Value=1/sqrt(3)
  Constant4 : Constant  Value=-1/sqrt(3)
  Product{,1..4} (5 alike) : Product
  Sum : Sum  Inputs=+++
  Sum1 : Sum
  Valpha : Outport
  Vbeta : Outport  Port=2
  wires:
  Product/1 -> Sum/1
  Constant1/1 -> Product1/1
  Product2/1 -> Sum/3
  Ua/1 -> Product/2
  Constant4/1 -> Product4/2
  Constant2/1 -> Product2/1
  Uc/1 -> Product4/1, Product2/2
  Constant/1 -> Product/1
  Sum/1 -> Valpha/1
  Product1/1 -> Sum/2
  Constant3/1 -> Product3/2
  Sum1/1 -> Vbeta/1
  Product3/1 -> Sum1/1
  Product4/1 -> Sum1/2
  Ub/1 -> Product3/1, Product1/2

== system Droop_GC/sm_computation/VSI 3/1_VSG control block/SRF PLL/Tpark ==
  Ualpha : Inport
  Ubeta : Inport  Port=2
  theta : Inport  Port=3
  Product{,1..3} (4 alike) : Product
  Sum : Sum
  Sum1 : Sum  Inputs=-+
  Trigonometric Function : Trigonometry
  Trigonometric Function1 : Trigonometry  Operator=cos
  Ud : Outport
  Uq : Outport  Port=2
  wires:
  Ualpha/1 -> Product/1, Product3/1
  Product3/1 -> Sum1/1
  Product1/1 -> Sum/2
  Trigonometric Function1/1 -> Product2/2, Product/2
  Ubeta/1 -> Product1/1, Product2/1
  Sum/1 -> Ud/1
  Product/1 -> Sum/1
  Trigonometric Function/1 -> Product3/2, Product1/2
  Sum1/1 -> Uq/1
  theta/1 -> Trigonometric Function1/1, Trigonometric Function/1
  Product2/1 -> Sum1/2

== system Droop_GC/sm_computation/VSI 3/1_VSG control block/SRF PLL1/SRF_PLL ==
  vq : Inport
  Center_Fre : Constant  Value=wn
  Center_Fre1 : Constant  Value=220*sqrt(2)
  Divide : Product  Inputs=*/
  Integrator : Integrator
  Integrator1 : Integrator
  Ki : Gain  Gain=Ki_pll
  Kp : Gain  Gain=Kp_pll
  Sum : Sum  Inputs=|++
  Sum1 : Sum  Inputs=++|
  wt : Outport
  wires:
  Divide/1 -> Ki/1, Kp/1
  Kp/1 -> Sum/1
  Ki/1 -> Integrator/1
  Integrator/1 -> Sum/2
  Sum/1 -> Sum1/2
  Sum1/1 -> Integrator1/1
  Integrator1/1 -> wt/1
  vq/1 -> Divide/1
  Center_Fre/1 -> Sum1/1
  Center_Fre1/1 -> Divide/2

== system Droop_GC/sm_computation/VSI 3/1_VSG control block/SRF PLL1/Tclark ==
  Ua : Inport
  Ub : Inport  Port=2
  Uc : Inport  Port=3
  Constant : Constant  Value=2/3
  Constant1 : Constant  Value=-1/3
  Constant2 : Constant  Value=-1/3
  Constant3 : Constant  Value=1/sqrt(3)
  Constant4 : Constant  Value=-1/sqrt(3)
  Product{,1..4} (5 alike) : Product
  Sum : Sum  Inputs=+++
  Sum1 : Sum
  Valpha : Outport
  Vbeta : Outport  Port=2
  wires:
  Product/1 -> Sum/1
  Constant1/1 -> Product1/1
  Product2/1 -> Sum/3
  Ua/1 -> Product/2
  Constant4/1 -> Product4/2
  Constant2/1 -> Product2/1
  Uc/1 -> Product4/1, Product2/2
  Constant/1 -> Product/1
  Sum/1 -> Valpha/1
  Product1/1 -> Sum/2
  Constant3/1 -> Product3/2
  Sum1/1 -> Vbeta/1
  Product3/1 -> Sum1/1
  Product4/1 -> Sum1/2
  Ub/1 -> Product3/1, Product1/2

== system Droop_GC/sm_computation/VSI 3/1_VSG control block/SRF PLL1/Tpark ==
  Ualpha : Inport
  Ubeta : Inport  Port=2
  theta : Inport  Port=3
  Product{,1..3} (4 alike) : Product
  Sum : Sum
  Sum1 : Sum  Inputs=-+
  Trigonometric Function : Trigonometry
  Trigonometric Function1 : Trigonometry  Operator=cos
  Ud : Outport
  Uq : Outport  Port=2
  wires:
  Ualpha/1 -> Product/1, Product3/1
  Product3/1 -> Sum1/1
  Product1/1 -> Sum/2
  Trigonometric Function1/1 -> Product2/2, Product/2
  Ubeta/1 -> Product1/1, Product2/1
  Sum/1 -> Ud/1
  Product/1 -> Sum/1
  Trigonometric Function/1 -> Product3/2, Product1/2
  Sum1/1 -> Uq/1
  theta/1 -> Trigonometric Function1/1, Trigonometric Function/1
  Product2/1 -> Sum1/2
